simulink model "System_dynamics"  (R2023b)
settings: Solver=FixedStepAuto  StartTime=0.0  StopTime=20  RelTol=1e-3
undefined symbols (not defined in the file or in its folder): x0
settings Model: Creator=ac140857  LastModifiedBy=fabioschneider
settings DataIOCC: SaveOutput=off  SaveTime=off

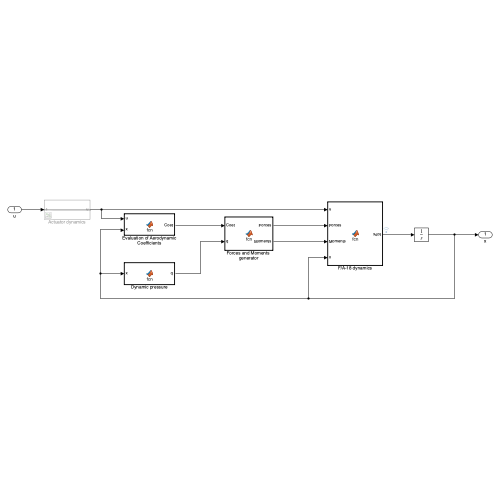
[thumbnail: Simulink's stored preview of the top-level diagram]
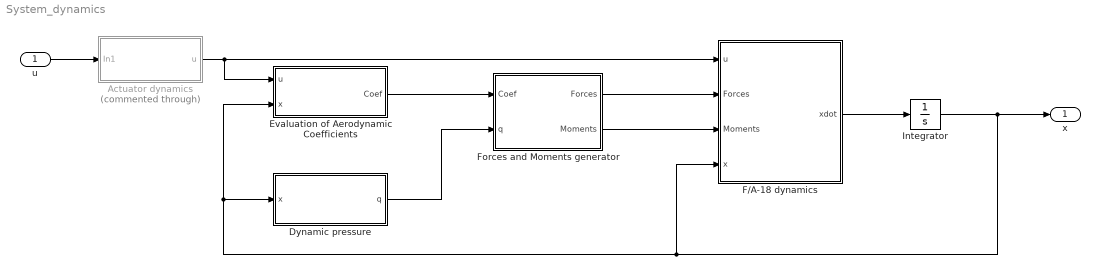
== system System_dynamics ==
  u : Inport  OutDataTypeStr=double  PortDimensions=4
  Actuator dynamics : Subsystem  Commented=through
  Dynamic pressure : MATLAB Function  TreatAsAtomicUnit=on
  Evaluation of Aerodynamic Coefficients : MATLAB Function  TreatAsAtomicUnit=on
  F/A-18 dynamics : MATLAB Function  TreatAsAtomicUnit=on
  Forces and Moments generator : MATLAB Function  TreatAsAtomicUnit=on
  Integrator : Integrator  InitialCondition=x0
  x : Outport  OutDataTypeStr=double  PortDimensions=[9 1]  SampleTime=0
  wires:
  F/A-18 dynamics/1(xdot) -> Integrator/1
  Integrator/1 -> Dynamic pressure/1(x), Evaluation of Aerodynamic Coefficients/2(x), F/A-18 dynamics/4(x), x/1
  Evaluation of Aerodynamic Coefficients/1(Coef) -> Forces and Moments generator/1(Coef)
  Dynamic pressure/1(q) -> Forces and Moments generator/2(q)
  Forces and Moments generator/1(Forces) -> F/A-18 dynamics/2(Forces)
  Forces and Moments generator/2(Moments) -> F/A-18 dynamics/3(Moments)
  u/1 -> Actuator dynamics/1(In1)
  Actuator dynamics/1(u) -> F/A-18 dynamics/1(u), Evaluation of Aerodynamic Coefficients/1(u)

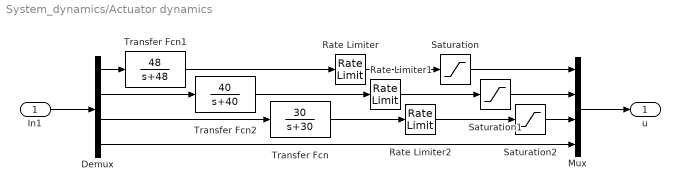
== system System_dynamics/Actuator dynamics ==
  In1 : Inport
  Demux : Demux
  Mux : Mux
  Rate Limiter : RateLimiter  RisingSlewLimit=100*pi/180  FallingSlewLimit=-100*pi/180  SampleTimeMode=inherited
  Rate Limiter1 : RateLimiter  RisingSlewLimit=100*pi/180  FallingSlewLimit=-100*pi/180  SampleTimeMode=inherited
  Rate Limiter2 : RateLimiter  RisingSlewLimit=40*pi/180  FallingSlewLimit=-40*pi/180  SampleTimeMode=inherited
  Saturation : Saturate  UpperLimit=45*pi/180  LowerLimit=-25*pi/180
  Saturation1 : Saturate  UpperLimit=45*pi/180  LowerLimit=-25*pi/180
  Saturation2 : Saturate  UpperLimit=10.5*pi/180  LowerLimit=-24*pi/180
  Transfer Fcn : TransferFcn  Numerator=[30]  Denominator=[1 30]
  Transfer Fcn1 : TransferFcn  Numerator=[48]  Denominator=[1 48]
  Transfer Fcn2 : TransferFcn  Numerator=[40]  Denominator=[1 40]
  u : Outport
  wires:
  Mux/1 -> u/1
  Rate Limiter2/1 -> Saturation2/1
  Rate Limiter1/1 -> Saturation1/1
  Rate Limiter/1 -> Saturation/1
  Saturation2/1 -> Mux/3
  Saturation1/1 -> Mux/2
  Saturation/1 -> Mux/1
  Demux/4 -> Mux/4
  Transfer Fcn/1 -> Rate Limiter2/1
  Demux/3 -> Transfer Fcn/1
  Demux/2 -> Transfer Fcn2/1
  Transfer Fcn2/1 -> Rate Limiter1/1
  Transfer Fcn1/1 -> Rate Limiter/1
  Demux/1 -> Transfer Fcn1/1
  In1/1 -> Demux/1

== matlab function System_dynamics/Evaluation of Aerodynamic Coefficients ==
  data: u input; Coef output; x input
function Coef = fcn(u, x)
    % INPUT:
    %   u = [ustab; urud; uail; uthr]
    %   x = [Velocity; sideslip_angle; angle_of_attack; rool_rate; pitch_rate; 
    %        yaw_rate; bank_angle; pitch_angle; yaw_angle]
    % OUTPUT:
    %   Coef = [Cm; Cl; Cn; CY; CL; CD];
    Coef = compute_coef(u,x);
end

== matlab function System_dynamics/F//A-18 dynamics ==
  data: u input; Forces input; Moments input; xdot output; x input
function xdot = fcn(u, Forces, Moments, x)

% u = [ustab; urud; uail; uthr]
% x = [Velocity; sideslip_angle; angle_of_attack; rool_rate; pitch_rate; 
% yaw_rate; bank_angle; pitch_angle; yaw_angle]
xdot = f(u, Forces, Moments, x); %Call the .m function
end

== matlab function System_dynamics/Forces and Moments generator ==
  data: Coef input; Forces output; q input; Moments output
function [Forces, Moments] = fcn(Coef, q)
    % INPUT:
    %   Coef = [Cm; Cl; Cn; CY; CL; CD];
    % OUTPUT:
    %   Forces = [D; L; Y]
    %   Moments = [l; M; n];
    [Forces, Moments] = compute_forces_moments(Coef, q);

end

== matlab function System_dynamics/Dynamic pressure ==
  data: x input; q output
function q = fcn(x)
    % INPUT:
    %   x = [Velocity; sideslip_angle; angle_of_attack; rool_rate; pitch_rate; 
    %        yaw_rate; bank_angle; pitch_angle; yaw_angle]
    % OUTPUT:
    %   q : dynamic pressure
    q = compute_dyn_pressure(x);

end
